simulink model "with_tf"  (R2020b)
settings: Solver=VariableStepAuto  StartTime=0.0  StopTime=10.0  RelTol=1e-3
settings Model: Creator=morro  LastModifiedBy=morro

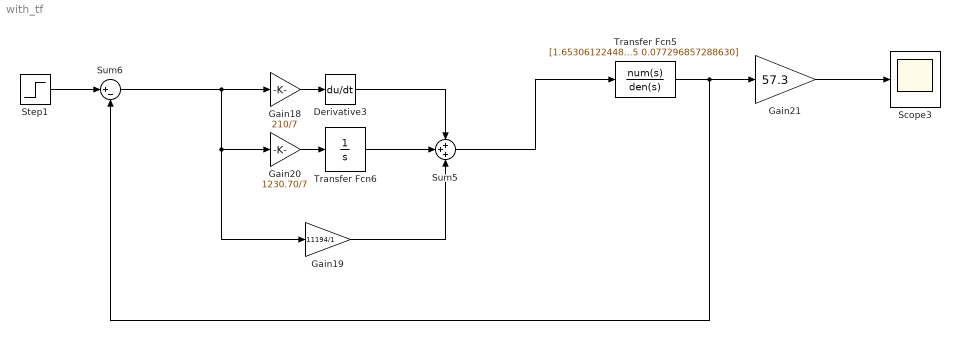
== system with_tf ==
  Derivative3 : Derivative
  Gain18 : Gain  Gain=210/7
  Gain19 : Gain  Gain=11194/1
  Gain20 : Gain  Gain=1230.70/7
  Gain21 : Gain  Gain=57.3
  Scope3 : Scope
  Step1 : Step  After=25/57.3  SampleTime=0
  Sum5 : Sum  Inputs=+++
  Sum6 : Sum  Inputs=|+-
  Transfer Fcn5 : TransferFcn  Numerator=[1.653061224489796e-06 0.009979591836735]  Denominator="[1.458000000000000e-12 1.760495641399417e-08  6.594754781341107e-05 0.077296857288630]"
  Transfer Fcn6 : TransferFcn  Denominator=[1 0]
  wires:
  Gain21/1 -> Scope3/1
  Transfer Fcn5/1 -> Sum6/2, Gain21/1
  Step1/1 -> Sum6/1
  Sum6/1 -> Gain20/1, Gain19/1, Gain18/1
  Gain19/1 -> Sum5/3
  Sum5/1 -> Transfer Fcn5/1
  Derivative3/1 -> Sum5/1
  Transfer Fcn6/1 -> Sum5/2
  Gain20/1 -> Transfer Fcn6/1
  Gain18/1 -> Derivative3/1
